simulink model "zadanienr3Simulink"  (R2024a)
settings: Solver=VariableStepAuto  StartTime=0.0  StopTime=10.0  RelTol=1e-3
values from neighbouring files (symbols this model uses):
  c = 400    [zadanie2TransmitancjaOperatorowa.m]
  M = 1000    [zadanie2TransmitancjaOperatorowa.m]
undefined symbols (not defined in the file or in its folder): a, F
settings Model: Creator=adasf  LastModifiedBy=adasf

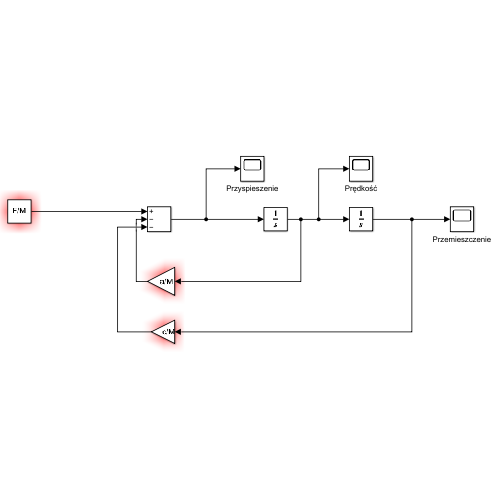
[thumbnail: Simulink's stored preview of the top-level diagram]
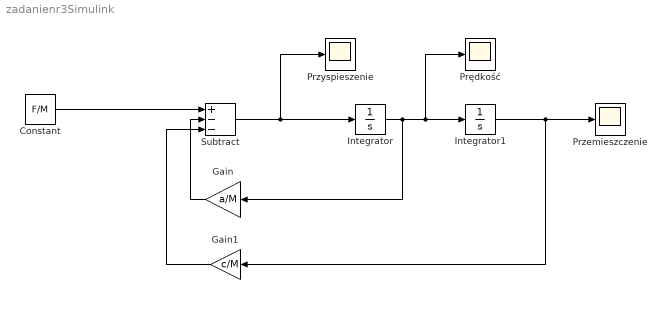
== system zadanienr3Simulink ==
  Constant : Constant  Value=F/M
  Gain : Gain  Gain=a/M
  Gain1 : Gain  Gain=c/M
  Integrator : Integrator
  Integrator1 : Integrator
  Przemieszczenie : Scope
  Przyspieszenie : Scope
  Prędkość : Scope
  Subtract : Sum  Inputs=+--
  wires:
  Constant/1 -> Subtract/1
  Gain/1 -> Subtract/2
  Gain1/1 -> Subtract/3
  Subtract/1 -> Integrator/1, Przyspieszenie/1
  Integrator/1 -> Gain/1, Integrator1/1, Prędkość/1
  Integrator1/1 -> Gain1/1, Przemieszczenie/1
